simulink model "k1visbs_oktm_20161207"  (Simulink 8.5)
settings: Solver=ode45  StartTime=0.0  StopTime=10.0  RelTol=1e-3
undefined symbols (not defined in the file): AC, FOUROSEM_OPLEV_DAMP_MASTER, SIXOSEM_F_STAGE_MASTER, SIXOSEM_F_WD_AC_MASTER
libraries: cdsEpicsOut x82, cdsFilt x57, cdsTP x36, cdsFiltCtrl x16, VIS_LIB x14, cdsMuxMatrix x13, cdsEpicsIn x10, cdsRms x6, STATE_BIO_MASTER x4, cdsEpicsBinIn x4, lockin x4, cdsFunctionCall x4
(part 1 of 8)
settings Model: Creator=keiko  LastModifiedBy=controls
settings DataIOCC: SignalLoggingSaveFormat=Dataset
settings OptimizationCC: ExpressionDepthLimit=128
settings DebuggingCC: UnderspecifiedInitializationDetection=Simplified  MergeDetectMultiDrivingBlocksExec=error  SolverPrmCheckMsg=warning  FcnCallInpInsideContextMsg=EnableAllAsError  StateNameClashWarn=none
settings GRTTargetCC: CombineOutputUpdateFcns=on  GRTInterface=off

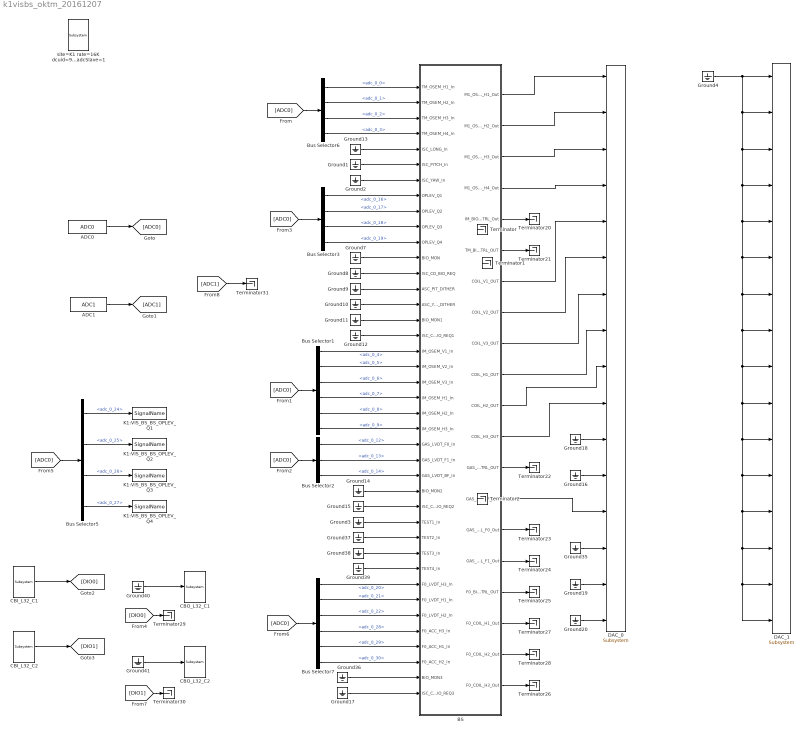
== system k1visbs_oktm_20161207 ==
  ADC0 : cdsAdcx0/ADC0  Tag=cdsAdc  Description=|
      | type-GSC_16AI64SSA
      | card_num=0
      settings: AttributesFormatString=%<Description>\n%<Tag>
  ADC1 : cdsAdcx1/ADC1  Tag=cdsAdc  Description=|
      | type-GSC_16AI64SSA
      | card_num=1
      settings: AttributesFormatString=%<Description>\n%<Tag>
  BS : Subsystem  Description=TYPEB MASTER  AncestorBlock=TYPEB_MASTER/TYPEB MASTER
      settings: AttributesFormatString=%<Description>
  Bus Selector1 : BusSelector  Description=ADC Selector  OutputSignals=adc_0_4,adc_0_5,adc_0_6,adc_0_7,adc_0_8,adc_0_9
      settings: AttributesFormatString=%<Description>
  Bus Selector2 : BusSelector  Description=ADC Selector  OutputSignals=adc_0_12,adc_0_13,adc_0_14
      settings: AttributesFormatString=%<Description>
  Bus Selector3 : BusSelector  Description=ADC Selector  OutputSignals=adc_0_16,adc_0_17,adc_0_18,adc_0_19
      settings: AttributesFormatString=%<Description>
  Bus Selector5 : BusSelector  Description=ADC Selector  OutputSignals=adc_0_24,adc_0_25,adc_0_26,adc_0_27
      settings: AttributesFormatString=%<Description>
  Bus Selector6 : BusSelector  Description=ADC Selector  OutputSignals=adc_0_0,adc_0_1,adc_0_2,adc_0_3
      settings: AttributesFormatString=%<Description>
  Bus Selector7 : BusSelector  Description=ADC Selector  OutputSignals=adc_0_20,adc_0_21,adc_0_22,adc_0_28,adc_0_29,adc_0_30
      settings: AttributesFormatString=%<Description>
  CBI_L32_C1 : cdsCDI64/Subsystem  Tag=cdsCDI64  Description=card_num=0
      settings: AttributesFormatString=%<Tag>\n%<Description>
  CBI_L32_C2 : cdsCDI64/Subsystem  Tag=cdsCDI64  Description=card_num=2
      settings: AttributesFormatString=%<Tag>\n%<Description>
  CBO_L32_C1 : cdsCDO64/Subsystem  Tag=cdsCDO64  Description=card_num=0
      settings: AttributesFormatString=%<Tag>\n%<Description>
  CBO_L32_C2 : cdsCDO64/Subsystem  Tag=cdsCDO64  Description=card_num=2
      settings: AttributesFormatString=%<Tag>\n%<Description>
  DAC_0 : dac/Subsystem  Description=|
      | type=GSC_16AO16,
      | card_num=0
      settings: AttributesFormatString=%<Description>
  DAC_1 : dac/Subsystem  Description=|
      | type=GSC_16AO16,
      | card_num=1
      settings: AttributesFormatString=%<Description>
  Ground{1..4,7..20,35..41} (25 alike) : Ground
  K1:VIS_BS_BS_OPLEV_Q{1..4} (4 alike) : cdsIPCx/SignalName  Tag=cdsIPCx_PCIE  Description=Inter-Process Communication via PCI Express network.
      settings: AttributesFormatString=%<Tag>
  Terminator{,1..2,20..31} (15 alike) : Terminator
  site=K1 rate=16K dcuid=96 host=k1pr2 specific_cpu=4 adcSlave=1 : cdsParameters/Subsystem  Tag=cdsParameters  Description=|
      | Purpose:                                                                                                                                                                                                                                
      | Provide system parameters to the FE code generator to properly configure the generated EPICS names, rep rate of the FE controller, and the Data Acquisition node ID for proper storage of data from this FE controller.                 
      |                                                                                                                                                                                                                                         
      | Useage:                                                                                                                                                                                                                                 
      | The part NAME field is used to identify the FE parameters. It must be of the form:                                                                                                                                                      
      | site=                                                                                                                                                                                                                                   
      | rate=                                                                                                                                                                                                                                   
      | dcuid=                                                                                                                                                                                                                                  
      |                                                                                                                                                                                                                                         
      | Where:                                                                                                                                                                                                                                  
      | site= argument may be H1, H2, L1, M1, G1, either as a single argument or multiple, for example site=H1,H2. These are the only names allowed. These will become the first two characters of all EPICS and signal names (for example G1:).
      |                                                                                                                                                                                                                                         
      | rate= may be 2K, 16K, 32K, or 64K                                                                                                                                                                                                       
      |                                                                                                                                                                                                                                         
      | dcuid= is site specific ie it must be unique at each site.
      settings: AttributesFormatString=%<Tag>
  wires:
  ADC0/1 -> [ADC0]
  [ADC0] -> Bus Selector6/1
  [ADC0] -> Bus Selector1/1
  Bus Selector6/1 -> BS/1(TM_OSEM_H1_In)  "<adc_0_0>"
  Bus Selector6/2 -> BS/2(TM_OSEM_H2_In)  "<adc_0_1>"
  Bus Selector6/3 -> BS/3(TM_OSEM_H3_In)  "<adc_0_2>"
  Bus Selector6/4 -> BS/4(TM_OSEM_H4_In)  "<adc_0_3>"
  Bus Selector3/4 -> BS/11(OPLEV_Q4)  "<adc_0_19>"
  Ground11/1 -> BS/16(BIO_MON1)
  Ground7/1 -> BS/12(BIO_MON)
  Ground2/1 -> BS/7(ISC_YAW_In)
  Ground8/1 -> BS/13(ISC_CD_BIO_REQ)
  Ground1/1 -> BS/6(ISC_PITCH_In)
  Ground12/1 -> BS/17(ISC_CD_BIO_REQ1)
  Ground13/1 -> BS/5(ISC_LONG_In)
  Bus Selector3/1 -> BS/8(OPLEV_Q1)  "<adc_0_16>"
  Bus Selector3/3 -> BS/10(OPLEV_Q3)  "<adc_0_18>"
  Bus Selector3/2 -> BS/9(OPLEV_Q2)  "<adc_0_17>"
  Ground10/1 -> BS/15(ASC_YAW_DITHER)
  Ground9/1 -> BS/14(ASC_PIT_DITHER)
  Bus Selector1/1 -> BS/18(IM_OSEM_V1_In)  "<adc_0_4>"
  Bus Selector1/2 -> BS/19(IM_OSEM_V2_In)  "<adc_0_5>"
  Bus Selector1/3 -> BS/20(IM_OSEM_V3_In)  "<adc_0_6>"
  Bus Selector1/4 -> BS/21(IM_OSEM_H1_In)  "<adc_0_7>"
  Bus Selector1/5 -> BS/22(IM_OSEM_H2_In)  "<adc_0_8>"
  Bus Selector1/6 -> BS/23(IM_OSEM_H3_In)  "<adc_0_9>"
  Ground14/1 -> BS/27(BIO_MON2)
  Ground15/1 -> BS/28(ISC_CD_BIO_REQ2)
  [ADC0] -> Bus Selector2/1
  Bus Selector2/1 -> BS/24(GAS_LVDT_F0_In)  "<adc_0_12>"
  [ADC0] -> Bus Selector3/1
  Ground3/1 -> BS/29(TEST1_In)
  [ADC0] -> Bus Selector5/1
  Bus Selector5/1 -> K1:VIS_BS_BS_OPLEV_Q1/1  "<adc_0_24>"
  Bus Selector5/2 -> K1:VIS_BS_BS_OPLEV_Q2/1  "<adc_0_25>"
  Bus Selector5/3 -> K1:VIS_BS_BS_OPLEV_Q3/1  "<adc_0_26>"
  Bus Selector5/4 -> K1:VIS_BS_BS_OPLEV_Q4/1  "<adc_0_27>"
  BS/1(M1_OSEM_H1_Out) -> DAC_0/1
  BS/2(M1_OSEM_H2_Out) -> DAC_0/2
  BS/3(M1_OSEM_H3_Out) -> DAC_0/3
  BS/4(M1_OSEM_H4_Out) -> DAC_0/4
  BS/5(IM_BIO_CTRL_Out) -> Terminator20/1
  BS/6(TM_BIO_CTRL_OUT) -> Terminator21/1
  Ground18/1 -> DAC_0/11
  Ground16/1 -> DAC_0/12
  Ground35/1 -> DAC_0/14
  Ground19/1 -> DAC_0/15
  Ground20/1 -> DAC_0/16
  BS/13(GAS_BIO_CTRL_OUT) -> Terminator22/1
  BS/14(GAS_COIL_BF_Out) -> DAC_0/13
  BS/10(COIL_H1_OUT) -> DAC_0/8
  BS/7(COIL_V1_OUT) -> DAC_0/5
  BS/9(COIL_V3_OUT) -> DAC_0/7
  BS/8(COIL_V2_OUT) -> DAC_0/6
  BS/11(COIL_H2_OUT) -> DAC_0/9
  BS/12(COIL_H3_OUT) -> DAC_0/10
  Ground17/1 -> BS/40(ISC_CD_BIO_REQ3)
  Bus Selector2/2 -> BS/25(GAS_LVDT_F1_In)  "<adc_0_13>"
  Bus Selector2/3 -> BS/26(GAS_LVDT_BF_In)  "<adc_0_14>"
  BS/15(GAS_COIL_F0_Out) -> Terminator23/1
  BS/16(GAS_COIL_F1_Out) -> Terminator24/1
  BS/17(F0_BIO_CTRL_OUT) -> Terminator25/1
  BS/20(F0_COIL_H3_Out) -> Terminator26/1
  BS/18(F0_COIL_H1_Out) -> Terminator27/1
  BS/19(F0_COIL_H2_Out) -> Terminator28/1
  [ADC0] -> Bus Selector7/1
  Ground36/1 -> BS/39(BIO_MON3)
  Ground37/1 -> BS/30(TEST2_In)
  Ground38/1 -> BS/31(TEST3_In)
  Ground39/1 -> BS/32(TEST4_In)
  Bus Selector7/1 -> BS/33(F0_LVDT_H3_In)  "<adc_0_20>"
  Bus Selector7/5 -> BS/37(F0_ACC_H1_In)  "<adc_0_29>"
  Bus Selector7/6 -> BS/38(F0_ACC_H2_In)  "<adc_0_30>"
  Bus Selector7/3 -> BS/35(F0_LVDT_H2_In)  "<adc_0_22>"
  Bus Selector7/2 -> BS/34(F0_LVDT_H1_In)  "<adc_0_21>"
  Bus Selector7/4 -> BS/36(F0_ACC_H3_In)  "<adc_0_28>"
  ADC1/1 -> [ADC1]
  CBI_L32_C1/1 -> [DIO0]
  CBI_L32_C2/1 -> [DIO1]
  Ground40/1 -> CBO_L32_C1/1
  Ground41/1 -> CBO_L32_C2/1
  [DIO0] -> Terminator29/1
  [DIO1] -> Terminator30/1
  [ADC1] -> Terminator31/1
  Ground4/1 -> DAC_1/6, DAC_1/16, DAC_1/15, DAC_1/14, DAC_1/13, DAC_1/12, DAC_1/11, DAC_1/10, DAC_1/9, DAC_1/8, DAC_1/7, DAC_1/5, DAC_1/4, DAC_1/3, DAC_1/2, DAC_1/1

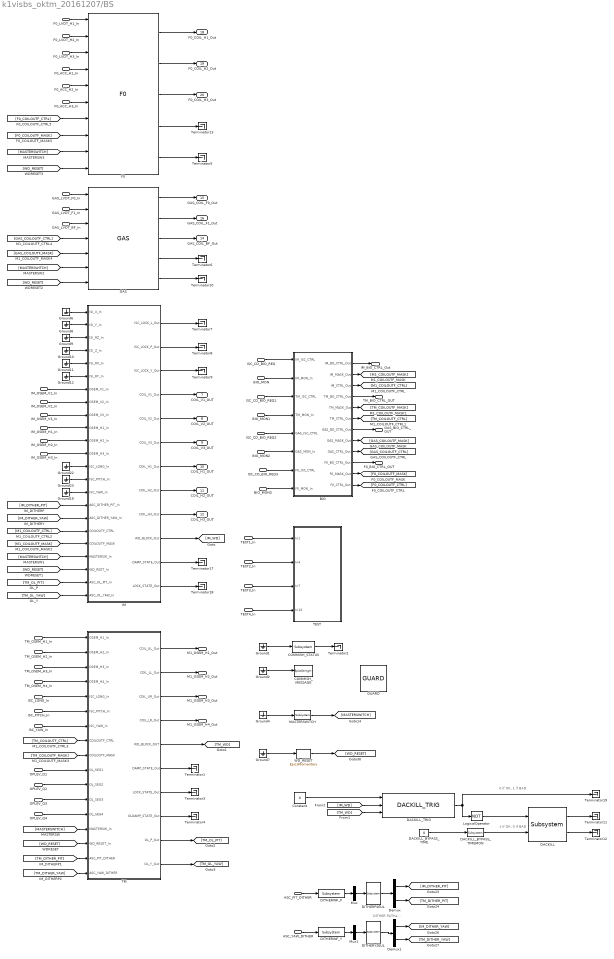
== system k1visbs_oktm_20161207/BS ==
  note: 1 if OK, 0 if BAD
  note: 0 if OK, 1 if BAD
  note: DITHER PATHs
      |
      |
      |
      |
      |
      |
      |
      |
      |
      |
      |
      |
      |
      |
      | .                                                                                                      .
  TM_OSEM_H1_In : Inport
  TM_OSEM_H2_In : Inport  Port=2
  TM_OSEM_H3_In : Inport  Port=3
  TM_OSEM_H4_In : Inport  Port=4
  ISC_LONG_In : Inport  Port=5
  ISC_PITCH_In : Inport  Port=6
  ISC_YAW_In : Inport  Port=7
  OPLEV_Q1 : Inport  Port=8
  OPLEV_Q2 : Inport  Port=9
  OPLEV_Q3 : Inport  Port=10
  OPLEV_Q4 : Inport  Port=11
  BIO_MON : Inport  Port=12
  ISC_CD_BIO_REQ : Inport  Port=13
  ASC_PIT_DITHER : Inport  Port=14
  ASC_YAW_DITHER : Inport  Port=15
  BIO_MON1 : Inport  Port=16
  ISC_CD_BIO_REQ1 : Inport  Port=17
  IM_OSEM_V1_In : Inport  Port=18
  IM_OSEM_V2_In : Inport  Port=19
  IM_OSEM_V3_In : Inport  Port=20
  IM_OSEM_H1_In : Inport  Port=21
  IM_OSEM_H2_In : Inport  Port=22
  IM_OSEM_H3_In : Inport  Port=23
  GAS_LVDT_F0_In : Inport  Port=24
  GAS_LVDT_F1_In : Inport  Port=25
  GAS_LVDT_BF_In : Inport  Port=26
  BIO_MON2 : Inport  Port=27
  ISC_CD_BIO_REQ2 : Inport  Port=28
  TEST1_In : Inport  Port=29
  TEST2_In : Inport  Port=30
  TEST3_In : Inport  Port=31
  TEST4_In : Inport  Port=32
  F0_LVDT_H3_In : Inport  Port=33
  F0_LVDT_H1_In : Inport  Port=34
  F0_LVDT_H2_In : Inport  Port=35
  F0_ACC_H3_In : Inport  Port=36
  F0_ACC_H1_In : Inport  Port=37
  F0_ACC_H2_In : Inport  Port=38
  BIO_MON3 : Inport  Port=39
  ISC_CD_BIO_REQ3 : Inport  Port=40
  BIO : Subsystem
  COMMISH_MESSAGE : cdsEpicsStringIn/EpicsStringIn  Tag=cdsEpicsStringIn  Description=cdsEpicsStringIn
      settings: AttributesFormatString=%<Tag>
  COMMISH_STATUS : cdsEpicsBinIn/Subsystem  Tag=cdsEpicsBinIn  Description=|
      | Purpose:                                                                            
      | Create an EPICS binary (0 or 1) input channel to the FE realtime controls.          
      |                                                                                     
      | Operation:                                                                          
      | Outputs value from an EPICS ai record. Value is binary input (bi Epics record type).
      |                                                                                     
      | Usage:                                                                              
      | Name the part with the desired EPICS channel name.
      settings: AttributesFormatString=%<Tag>
  Constant : Constant  Value=0
  DACKILL : cdsDacKill/Subsystem  Description=cdsDacKill
      settings: AttributesFormatString=%<Description>
  DACKILL_BYPASS_TIME : Constant  Value=0
  DACKILL_BYPASS_TIMEMON : cdsEpicsOut/Subsystem  Tag=cdsEpicsOutput  Description=|
      | Purpose:                                          
      | Output a FE signal to an EPICS channel.           
      |                                                   
      | Operation:                                        
      | Takes input value and passes it to EPICS record.  
      |                                                   
      | Usage:                                            
      | Name the part with the desired EPICS rrecord name.
      settings: AttributesFormatString=%<Tag>
  DACKILL_TRIG : VIS_LIB/DACKILL_TRIG
  DITHERINF_P : cdsFilt/Subsystem  Tag=cdsFilt  Description=|
      | Purpose:                                                                                                                                                                                                                                  
      | Standard CDS IIR filter module.                                                                                                                                                                                                           
      |                                                                                                                                                                                                                                           
      | Operation:                                                                                                                                                                                                                                
      | Consists of 10 second order section IIR filters, plus a ramped gain stage. In FE code, also provides pre-defined test points and excitation channel inputs. The filter coefficients are defined in the LIGO system using the 'foton' tool.
      |                                                                                                                                                                                                                                           
      | Usage:                                                                                                                                                                                                                                    
      | Name the part with the desired filter module name.
      settings: AttributesFormatString=%<Tag>
  DITHERINF_Y : cdsFilt/Subsystem  Tag=cdsFilt  Description=|
      | Purpose:                                                                                                                                                                                                                                  
      | Standard CDS IIR filter module.                                                                                                                                                                                                           
      |                                                                                                                                                                                                                                           
      | Operation:                                                                                                                                                                                                                                
      | Consists of 10 second order section IIR filters, plus a ramped gain stage. In FE code, also provides pre-defined test points and excitation channel inputs. The filter coefficients are defined in the LIGO system using the 'foton' tool.
      |                                                                                                                                                                                                                                           
      | Usage:                                                                                                                                                                                                                                    
      | Name the part with the desired filter module name.
      settings: AttributesFormatString=%<Tag>
  DITHERP2EUL : cdsMuxMatrix/Subsystem  Tag=cdsMuxMatrix  Description=Any size matrix. Inputs and outputs must be connected using Mux and Demux parts.
      settings: AttributesFormatString=%<Tag>
  DITHERY2EUL : cdsMuxMatrix/Subsystem  Tag=cdsMuxMatrix  Description=Any size matrix. Inputs and outputs must be connected using Mux and Demux parts.
      settings: AttributesFormatString=%<Tag>
  Demux : Demux  Outputs=2
  Demux1 : Demux  Outputs=2
  F0 : F0_MASTER/F0
  GAS : GAS_TYPEB_MASTER/GAS  Tag=GAS_TYPEB_MASTER  Description=GAS_TYPEB_MASTER
  GUARD : ISC_common/GUARD
  Ground{1..2,4,6..12,19,22..23} (13 alike) : Ground
  IM : Subsystem  Description=SIXOSEMSTAGE_FACE_MASTER  AncestorBlock=SIXOSEM_F_STAGE_MASTER/SIXOSEM_F_STAGE_MASTER
  LogicalOperator : Logic  Operator=NOT  AllPortsSameDT=off  OutDataTypeStr=boolean
  MASTERSWITCH : cdsEpicsBinIn/Subsystem  Tag=cdsEpicsBinIn  Description=|
      | Purpose:                                                                            
      | Create an EPICS binary (0 or 1) input channel to the FE realtime controls.          
      |                                                                                     
      | Operation:                                                                          
      | Outputs value from an EPICS ai record. Value is binary input (bi Epics record type).
      |                                                                                     
      | Usage:                                                                              
      | Name the part with the desired EPICS channel name.
      settings: AttributesFormatString=%<Tag>
  Mux : Mux  Inputs=1
  Mux1 : Mux  Inputs=1
  TEST : Subsystem
  TM : Subsystem  AncestorBlock=FOUROSEM_OPLEV_DAMP_MASTER/FOUROSEM_OPLEV_DAMP_MASTER
  Terminator{1..13,17..19} (16 alike) : Terminator
  WD_RESET : cdsEpicsMomentary/EpicsMomentary  Tag=cdsEpicsMomentary
      settings: AttributesFormatString=%<Tag>
  M1_OSEM_H1_Out : Outport
  M1_OSEM_H2_Out : Outport  Port=2
  M1_OSEM_H3_Out : Outport  Port=3
  M1_OSEM_H4_Out : Outport  Port=4
  IM_BIO_CTRL_Out : Outport  Port=5
  TM_BIO_CTRL_OUT : Outport  Port=6
  COIL_V1_OUT : Outport  Port=7
  COIL_V2_OUT : Outport  Port=8
  COIL_V3_OUT : Outport  Port=9
  COIL_H1_OUT : Outport  Port=10
  COIL_H2_OUT : Outport  Port=11
  COIL_H3_OUT : Outport  Port=12
  GAS_BIO_CTRL_OUT : Outport  Port=13
  GAS_COIL_BF_Out : Outport  Port=14
  GAS_COIL_F0_Out : Outport  Port=15
  GAS_COIL_F1_Out : Outport  Port=16
  F0_BIO_CTRL_OUT : Outport  Port=17
  F0_COIL_H1_Out : Outport  Port=18
  F0_COIL_H2_Out : Outport  Port=19
  F0_COIL_H3_Out : Outport  Port=20
  wires:
  F0_ACC_H2_In/1 -> F0/5
  F0_LVDT_H3_In/1 -> F0/3
  F0_LVDT_H1_In/1 -> F0/1
  F0_ACC_H1_In/1 -> F0/4
  F0_LVDT_H2_In/1 -> F0/2
  F0_ACC_H3_In/1 -> F0/6
  GAS/2 -> GAS_COIL_F1_Out/1
  GAS/1 -> GAS_COIL_F0_Out/1
  GAS_LVDT_F0_In/1 -> GAS/1
  GAS_LVDT_F1_In/1 -> GAS/2
  TM/10(OL_Y_Out) -> [TM_OL_YAW]
  TM/9(OL_P_Out) -> [TM_OL_PIT]
  [TM_OL_YAW] -> IM/23(ASC_OL_YAW_In)
  [TM_OL_PIT] -> IM/22(ASC_OL_PIT_In)
  [WD_RESET] -> IM/21(WD_RSET_In)
  [MASTERSWITCH] -> IM/20(MASTERSW_In)
  [M1_COILOUTF_MASK] -> IM/19(COILOUTF_MASK)
  [IM_DITHER_YAW] -> IM/17(ASC_DITHER_YAW_In)
  [IM_DITHER_PIT] -> IM/16(ASC_DITHER_PIT_In)
  [M1_COILOUTF_CTRL] -> IM/18(COILOUTF_CTRL)
  [IM_WD] -> DACKILL_TRIG/2
  DACKILL/2 -> Terminator12/1
  DACKILL/1 -> Terminator11/1
  DACKILL_BYPASS_TIME/1 -> DACKILL_BYPASS_TIMEMON/1
  DACKILL_BYPASS_TIMEMON/1 -> DACKILL/2
  LogicalOperator/1 -> DACKILL/1
  DACKILL_TRIG/1 -> LogicalOperator/1, Terminator19/1
  Constant/1 -> DACKILL_TRIG/1
  [TM_WD] -> DACKILL_TRIG/3
  TM/1(COIL_UL_Out) -> M1_OSEM_H1_Out/1
  TEST4_In/1 -> TEST/4(In10)
  TEST1_In/1 -> TEST/1(In1)
  TEST2_In/1 -> TEST/2(In4)
  TEST3_In/1 -> TEST/3(In7)
  GAS/5 -> Terminator10/1
  GAS/4 -> Terminator6/1
  GAS/3 -> GAS_COIL_BF_Out/1
  [WD_RESET] -> GAS/7
  [MASTERSWITCH] -> GAS/6
  [GAS_COILOUTF_MASK] -> GAS/5
  BIO_MON2/1 -> BIO/6(GAS_MON_In)
  ISC_CD_BIO_REQ2/1 -> BIO/5(GAS_ISC_CTRL)
  BIO/9(GAS_CTRL_Out) -> [GAS_COILOUTF_CTRL]
  BIO/8(GAS_MASK_Out) -> [GAS_COILOUTF_MASK]
  BIO/7(GAS_BO_CTRL_Out) -> GAS_BIO_CTRL_OUT/1
  [GAS_COILOUTF_CTRL] -> GAS/4
  GAS_LVDT_BF_In/1 -> GAS/3
  IM/9(COIL_H3_Out) -> COIL_H3_OUT/1
  IM/8(COIL_H2_Out) -> COIL_H2_OUT/1
  IM/7(COIL_H1_Out) -> COIL_H1_OUT/1
  IM/6(COIL_V3_Out) -> COIL_V3_OUT/1
  IM/5(COIL_V2_Out) -> COIL_V2_OUT/1
  IM/4(COIL_V1_Out) -> COIL_V1_OUT/1
  IM_OSEM_H1_In/1 -> IM/10(OSEM_H1_In)
  IM_OSEM_H2_In/1 -> IM/11(OSEM_H2_In)
  IM_OSEM_H3_In/1 -> IM/12(OSEM_H3_In)
  IM_OSEM_V1_In/1 -> IM/7(OSEM_V1_In)
  IM_OSEM_V2_In/1 -> IM/8(OSEM_V2_In)
  IM_OSEM_V3_In/1 -> IM/9(OSEM_V3_In)
  IM/12(LOCK_STATE_Out) -> Terminator18/1
  IM/3(ISC_LOCK_Y_Out) -> Terminator9/1
  IM/2(ISC_LOCK_P_Out) -> Terminator8/1
  IM/11(DAMP_STATE_Out) -> Terminator17/1
  IM/10(WD_BLOCK_Out) -> [IM_WD]
  IM/1(ISC_LOCK_L_Out) -> Terminator7/1
  Ground19/1 -> IM/15(ISC_YAW_In)
  Ground23/1 -> IM/14(ISC_PITCH_In)
  Ground12/1 -> IM/6(ISI_RY_In)
  Ground10/1 -> IM/4(ISI_Z_In)
  Ground22/1 -> IM/13(ISC_LONG_In)
  Ground8/1 -> IM/2(ISI_Y_In)
  Ground6/1 -> IM/1(ISI_X_In)
  Ground11/1 -> IM/5(ISI_RX_In)
  Ground9/1 -> IM/3(ISI_RZ_In)
  [TM_DITHER_YAW] -> TM/17(ASC_YAW_DITHER)
  [TM_DITHER_PIT] -> TM/16(ASC_PIT_DITHER)
  DITHERINF_Y/1 -> Mux1/1
  DITHERINF_P/1 -> Mux/1
  Demux1/2 -> [TM_DITHER_YAW]
  Demux1/1 -> [IM_DITHER_YAW]
  Demux/2 -> [TM_DITHER_PIT]
  Demux/1 -> [IM_DITHER_PIT]
  DITHERY2EUL/1 -> Demux1/1
  Mux1/1 -> DITHERY2EUL/1
  ASC_PIT_DITHER/1 -> DITHERINF_P/1
  DITHERP2EUL/1 -> Demux/1
  Mux/1 -> DITHERP2EUL/1
  ASC_YAW_DITHER/1 -> DITHERINF_Y/1
  Ground1/1 -> COMMISH_STATUS/1
  COMMISH_STATUS/1 -> Terminator2/1
  Ground2/1 -> COMMISH_MESSAGE/1
  TM_OSEM_H1_In/1 -> TM/1(OSEM_H1_In)
  TM_OSEM_H2_In/1 -> TM/2(OSEM_H2_In)
  TM_OSEM_H3_In/1 -> TM/3(OSEM_H3_In)
  TM_OSEM_H4_In/1 -> TM/4(OSEM_H4_In)
  ISC_LONG_In/1 -> TM/5(ISC_LONG_In)
  TM/5(WD_BLOCK_OUT) -> [TM_WD]
  BIO/3(IM_CTRL_Out) -> [M1_COILOUTF_CTRL]
  BIO/2(IM_MASK_Out) -> [M1_COILOUTF_MASK]
  BIO/1(IM_BO_CTRL_Out) -> IM_BIO_CTRL_Out/1
  TM/2(COIL_LL_Out) -> M1_OSEM_H2_Out/1
  TM/3(COIL_UR_Out) -> M1_OSEM_H3_Out/1
  TM/4(COIL_LR_Out) -> M1_OSEM_H4_Out/1
  BIO_MON/1 -> BIO/2(IM_MON_In)
  ISC_CD_BIO_REQ/1 -> BIO/1(IM_ISC_CTRL)
  MASTERSWITCH/1 -> [MASTERSWITCH]
  Ground4/1 -> MASTERSWITCH/1
  OPLEV_Q1/1 -> TM/10(OL_SEG1)
  OPLEV_Q2/1 -> TM/11(OL_SEG2)
  OPLEV_Q3/1 -> TM/12(OL_SEG3)
  ISC_PITCH_In/1 -> TM/6(ISC_PITCH_In)
  ISC_YAW_In/1 -> TM/7(ISC_YAW_In)
  OPLEV_Q4/1 -> TM/13(OL_SEG4)
  [MASTERSWITCH] -> TM/14(MASTERSW_In)
  TM/8(OLDAMP_STATE_Out) -> Terminator4/1
  TM/7(LOCK_STATE_Out) -> Terminator3/1
  TM/6(DAMP_STATE_Out) -> Terminator1/1
  Ground7/1 -> WD_RESET/1
  WD_RESET/1 -> [WD_RESET]
  [WD_RESET] -> TM/15(WD_RESET_In)
  BIO_MON1/1 -> BIO/4(TM_MON_In)
  ISC_CD_BIO_REQ1/1 -> BIO/3(TM_ISC_CTRL)
  BIO/5(TM_MASK_Out) -> [TM_COILOUTF_MASK]
  BIO/6(TM_CTRL_Out) -> [TM_COILOUTF_CTRL]
  BIO/4(TM_BO_CTRL_Out) -> TM_BIO_CTRL_OUT/1
  [TM_COILOUTF_CTRL] -> TM/8(COILOUTF_CTRL)
  [TM_COILOUTF_MASK] -> TM/9(COILOUTF_MASK)
  [MASTERSWITCH] -> F0/9
  [WD_RESET] -> F0/10
  BIO/11(F0_MASK_Out) -> [F0_COILOUTF_MASK]
  BIO/12(F0_CTRL_Out) -> [F0_COILOUTF_CTRL]
  BIO/10(F0_BO_CTRL_Out) -> F0_BIO_CTRL_OUT/1
  BIO_MON3/1 -> BIO/8(F0_MON_In)
  ISC_CD_BIO_REQ3/1 -> BIO/7(F0_ISC_CTRL)
  [F0_COILOUTF_CTRL] -> F0/7
  [F0_COILOUTF_MASK] -> F0/8
  F0/5 -> Terminator5/1
  F0/4 -> Terminator13/1
  F0/3 -> F0_COIL_H3_Out/1
  F0/2 -> F0_COIL_H2_Out/1
  F0/1 -> F0_COIL_H1_Out/1

== system k1visbs_oktm_20161207/BS/BIO ==
  note: 12 Bit Word
  note: 12 Bit Word
  note: 12 Bit Word
  note: 12 Bit Word
  note: 12 Bit Word
  note: 12 Bit Word
  note: 12 Bit Word
  note: 12 Bit Word
  IM_ISC_CTRL : Inport
  IM_MON_In : Inport  Port=2
  TM_ISC_CTRL : Inport  Port=3
  TM_MON_In : Inport  Port=4
  GAS_ISC_CTRL : Inport  Port=5
  GAS_MON_In : Inport  Port=6
  F0_ISC_CTRL : Inport  Port=7
  F0_MON_In : Inport  Port=8
  F0 : STATE_BIO_MASTER/TACQ_BIO_MASTER
  GAS : STATE_BIO_MASTER/TACQ_BIO_MASTER
  IM : STATE_BIO_MASTER/TOP_BIO_MASTER
  TM : STATE_BIO_MASTER/TACQ_BIO_MASTER
  IM_BO_CTRL_Out : Outport
  IM_MASK_Out : Outport  Port=2
  IM_CTRL_Out : Outport  Port=3
  TM_BO_CTRL_Out : Outport  Port=4
  TM_MASK_Out : Outport  Port=5
  TM_CTRL_Out : Outport  Port=6
  GAS_BO_CTRL_Out : Outport  Port=7
  GAS_MASK_Out : Outport  Port=8
  GAS_CTRL_Out : Outport  Port=9
  F0_BO_CTRL_Out : Outport  Port=10
  F0_MASK_Out : Outport  Port=11
  F0_CTRL_Out : Outport  Port=12
  wires:
  GAS/2 -> GAS_CTRL_Out/1
  GAS/1 -> GAS_MASK_Out/1
  GAS/3 -> GAS_BO_CTRL_Out/1
  GAS_MON_In/1 -> GAS/2
  GAS_ISC_CTRL/1 -> GAS/1
  IM/2 -> IM_CTRL_Out/1
  IM/1 -> IM_MASK_Out/1
  IM/3 -> IM_BO_CTRL_Out/1
  IM_MON_In/1 -> IM/2
  IM_ISC_CTRL/1 -> IM/1
  TM/2 -> TM_CTRL_Out/1
  TM/1 -> TM_MASK_Out/1
  TM/3 -> TM_BO_CTRL_Out/1
  TM_MON_In/1 -> TM/2
  TM_ISC_CTRL/1 -> TM/1
  F0/2 -> F0_CTRL_Out/1
  F0/1 -> F0_MASK_Out/1
  F0/3 -> F0_BO_CTRL_Out/1
  F0_MON_In/1 -> F0/2
  F0_ISC_CTRL/1 -> F0/1

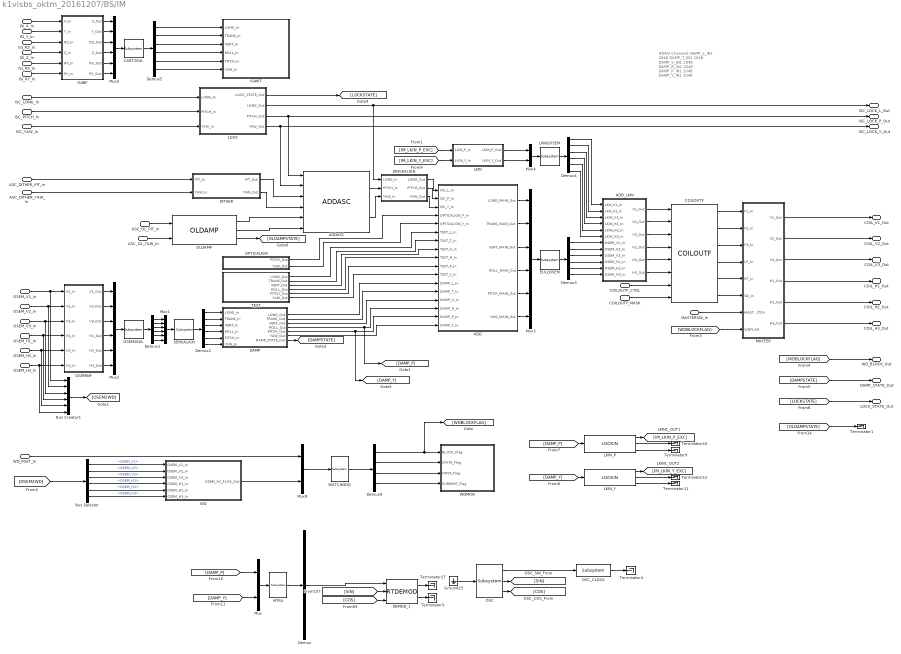
== system k1visbs_oktm_20161207/BS/IM ==
  note: #DAQ Channels
      | DAMP_L_IN1 2048
      | DAMP_T_IN1 2048
      | DAMP_V_IN1 2048
      | DAMP_R_IN1 2048
      | DAMP_P_IN1 2048
      | DAMP_Y_IN1 2048
  ISI_X_In : Inport
  ISI_Y_In : Inport  Port=2
  ISI_RZ_In : Inport  Port=3
  ISI_Z_In : Inport  Port=4
  ISI_RX_In : Inport  Port=5
  ISI_RY_In : Inport  Port=6
  OSEM_V1_In : Inport  Port=7
  OSEM_V2_In : Inport  Port=8
  OSEM_V3_In : Inport  Port=9
  OSEM_H1_In : Inport  Port=10
  OSEM_H2_In : Inport  Port=11
  OSEM_H3_In : Inport  Port=12
  ISC_LONG_In : Inport  Port=13
  ISC_PITCH_In : Inport  Port=14
  ISC_YAW_In : Inport  Port=15
  ASC_DITHER_PIT_In : Inport  Port=16
  ASC_DITHER_YAW_In : Inport  Port=17
  COILOUTF_CTRL : Inport  Port=18
  COILOUTF_MASK : Inport  Port=19
  MASTERSW_In : Inport  Port=20
  WD_RSET_In : Inport  Port=21
  ASC_OL_PIT_In : Inport  Port=22
  ASC_OL_YAW_In : Inport  Port=23
  ADD : Subsystem
  ADDASC : VIS_LIB/ADDASC
  ADD_LKIN : Subsystem
  Bus Creator1 : BusCreator  Inputs='OSEM_V1','OSEM_V2','OSEM_V3','OSEM_H1','OSEM_H2','OSEM_H3'
  Bus Selector : BusSelector  OutputSignals=OSEM_V1,OSEM_V2,OSEM_V3,OSEM_H1,OSEM_H2,OSEM_H3
  CART2EUL : cdsMuxMatrix/Subsystem  Tag=cdsMuxMatrix  Description=Any size matrix. Inputs and outputs must be connected using Mux and Demux parts.
      settings: AttributesFormatString=%<Tag>
  COILOUTF : SIXOSEM_F_COILOUTF_MASTER/COILOUTF
  DAMP : Subsystem
  DEMOD_1 : rtdemod/RTDEMOD  Tag=top_names
  DITHER : Subsystem
  DRIVEALIGN : Subsystem
  Demux : Demux  Outputs=1
  Demux{1..5} (5 alike) : Demux  Outputs=6
  Demux9 : Demux
  EUL2OSEM : cdsMuxMatrix/Subsystem  Tag=cdsMuxMatrix  Description=Any size matrix. Inputs and outputs must be connected using Mux and Demux parts.
      settings: AttributesFormatString=%<Tag>
  Ground23 : Ground
  ISIINF : Subsystem
  ISIWIT : Subsystem
  LKIN : Subsystem
  LKIN2OSEM : cdsMuxMatrix/Subsystem  Tag=cdsMuxMatrix  Description=Any size matrix. Inputs and outputs must be connected using Mux and Demux parts.
      settings: AttributesFormatString=%<Tag>
  LKIN_P : lockin/LOCKIN  Description=ADL=LOCKIN.adl
      settings: AttributesFormatString=%<Tag>
  LKIN_Y : lockin/LOCKIN  Description=ADL=LOCKIN.adl
      settings: AttributesFormatString=%<Tag>
  LOCK : Subsystem
  MASTER : Subsystem
  MTRX : cdsMuxMatrix/Subsystem  Tag=cdsMuxMatrix  Description=Any size matrix. Inputs and outputs must be connected using Mux and Demux parts.
      settings: AttributesFormatString=%<Tag>
  Mux : Mux  Inputs=2
  Mux{1..3,5} (4 alike) : Mux  Inputs=6
  Mux4 : Mux  Inputs=2
  Mux9 : Mux  Inputs=2
  OLDAMP : VIS_LIB/OLDAMP
  OPTICALIGN : Subsystem
  OSC : cdsOsc/Subsystem  Tag=cdsOsc  Description=Oscillator
      settings: AttributesFormatString=%<Tag>
  OSC_CLOCK : cdsEpicsOut/Subsystem  Tag=cdsEpicsOutput  Description=|
      | Purpose:                                          
      | Output a FE signal to an EPICS channel.           
      |                                                   
      | Operation:                                        
      | Takes input value and passes it to EPICS record.  
      |                                                   
      | Usage:                                            
      | Name the part with the desired EPICS rrecord name.
      settings: AttributesFormatString=%<Tag>
  OSEM2EUL : cdsMuxMatrix/Subsystem  Tag=cdsMuxMatrix  Description=Any size matrix. Inputs and outputs must be connected using Mux and Demux parts.
      settings: AttributesFormatString=%<Tag>
  OSEMINF : Subsystem
  SENSALIGN : cdsMuxMatrix/Subsystem  Tag=cdsMuxMatrix  Description=Any size matrix. Inputs and outputs must be connected using Mux and Demux parts.
      settings: AttributesFormatString=%<Tag>
  TEST : Subsystem
  Terminator{1,3..4,9..12,27} (8 alike) : Terminator
  WATCHDOG : cdsFunctionCall/Subsystem  Tag=cdsFunctionCall  Description=inline OSEMWATCHDOG /opt/rtcds/userapps/release/vis/common/src/WATCHDOG.c
      settings: AttributesFormatString=%<Tag>\n%<Description>
  WD : Subsystem
  WDMON : Subsystem
  ISC_LOCK_L_Out : Outport
  ISC_LOCK_P_Out : Outport  Port=2
  ISC_LOCK_Y_Out : Outport  Port=3
  COIL_V1_Out : Outport  Port=4
  COIL_V2_Out : Outport  Port=5
  COIL_V3_Out : Outport  Port=6
  COIL_H1_Out : Outport  Port=7
  COIL_H2_Out : Outport  Port=8
  COIL_H3_Out : Outport  Port=9
  WD_BLOCK_Out : Outport  Port=10
  DAMP_STATE_Out : Outport  Port=11
  LOCK_STATE_Out : Outport  Port=12
  wires:
  [OLDAMPSTATE] -> Terminator1/1
  ASC_OL_PIT_In/1 -> OLDAMP/1
  ASC_OL_YAW_In/1 -> OLDAMP/2
  OLDAMP/1 -> ADDASC/5
  OLDAMP/2 -> ADDASC/6
  OLDAMP/3 -> [OLDAMPSTATE]
  Mux/1 -> MTRX/1
  MTRX/1 -> Demux/1
  Demux/1 -> DEMOD_1/1
  [SIN] -> DEMOD_1/2
  [COS] -> DEMOD_1/3
  DEMOD_1/1 -> Terminator27/1
  DEMOD_1/2 -> Terminator3/1
  Ground23/1 -> OSC/1
  OSC/1 -> OSC_CLOCK/1
  OSC_CLOCK/1 -> Terminator4/1
  OSC/2 -> [SIN]
  OSC/3 -> [COS]
  [DAMP_P] -> Mux/1
  [DAMP_Y] -> Mux/2
  [DAMP_Y] -> LKIN_Y/1
  [DAMP_P] -> LKIN_P/1
  [IM_LKIN_Y_EXC] -> LKIN/2(LKIN_Y_In)
  [IM_LKIN_P_EXC] -> LKIN/1(LKIN_P_In)
  LKIN_Y/3 -> Terminator11/1
  LKIN_Y/2 -> Terminator12/1
  LKIN_Y/1 -> [IM_LKIN_Y_EXC]
  LKIN_P/1 -> [IM_LKIN_P_EXC]
  LKIN_P/3 -> Terminator9/1
  LKIN_P/2 -> Terminator10/1
  DAMP/1(LONG_Out) -> ADD/12(DAMP_L_In)
  DAMP/2(TRANS_Out) -> ADD/13(DAMP_T_In)
  DAMP/3(VERT_Out) -> ADD/14(DAMP_V_In)
  DAMP/4(ROLL_Out) -> ADD/15(DAMP_R_In), [DAMP_P]
  DAMP/5(PITCH_Out) -> ADD/16(DAMP_P_In), [DAMP_Y]
  DAMP/6(YAW_Out) -> ADD/17(DAMP_Y_In)
  TEST/1(LONG_Out) -> ADD/6(TEST_L_In)
  TEST/2(TRANS_Out) -> ADD/7(TEST_T_In)
  TEST/3(VERT_Out) -> ADD/8(TEST_V_In)
  TEST/4(ROLL_Out) -> ADD/9(TEST_R_In)
  TEST/5(PITCH_Out) -> ADD/10(TEST_P_In)
  TEST/6(YAW_Out) -> ADD/11(TEST_Y_In)
  OPTICALIGN/1(PITCH_Out) -> ADD/4(OPTICALIGN_P_In)
  OPTICALIGN/2(YAW_Out) -> ADD/5(OPTICALIGN_Y_In)
  DITHER/1(PIT_Out) -> ADDASC/3
  DITHER/2(YAW_Out) -> ADDASC/4
  ASC_DITHER_PIT_In/1 -> DITHER/1(PIT_In)
  ASC_DITHER_YAW_In/1 -> DITHER/2(YAW_In)
  ADDASC/2 -> DRIVEALIGN/3(YAW_In)
  ADDASC/1 -> DRIVEALIGN/2(PITCH_In)
  DRIVEALIGN/1(LONG_Out) -> ADD/1(ISC_L_In)
  DRIVEALIGN/2(PITCH_Out) -> ADD/2(ISC_P_In)
  DRIVEALIGN/3(YAW_Out) -> ADD/3(ISC_Y_In)
  LOCK/4(YAW_Out) -> ISC_LOCK_Y_Out/1, ADDASC/2
  LOCK/3(PITCH_Out) -> ISC_LOCK_P_Out/1, ADDASC/1
  LOCK/2(LONG_Out) -> ISC_LOCK_L_Out/1, DRIVEALIGN/1(LONG_In)
  WD_RSET_In/1 -> Mux9/1
  WD/1(OSEM_AC_FLAG_Out) -> Mux9/2
  LKIN/2(LKIN_Y_Out) -> Mux4/2
  COILOUTF_CTRL/1 -> COILOUTF/7
  COILOUTF_MASK/1 -> COILOUTF/8
  MASTERSW_In/1 -> MASTER/7(MASTERSWITCH)
  Demux3/6 -> ADD_LKIN/12(OSEM_H3_In)
  Demux3/5 -> ADD_LKIN/11(OSEM_H2_In)
  Demux3/4 -> ADD_LKIN/10(OSEM_H1_In)
  Demux3/3 -> ADD_LKIN/9(OSEM_V3_In)
  Demux3/2 -> ADD_LKIN/8(OSEM_V2_In)
  Demux3/1 -> ADD_LKIN/7(OSEM_V1_In)
  Demux4/6 -> ADD_LKIN/6(LKIN_H3_In)
  Demux4/5 -> ADD_LKIN/5(LKIN_H2_In)
  Demux4/4 -> ADD_LKIN/4(LKIN_H1_In)
  Demux4/3 -> ADD_LKIN/3(LKIN_V3_In)
  Demux4/2 -> ADD_LKIN/2(LKN_V2_In)
  Demux4/1 -> ADD_LKIN/1(LKN_V1_In)
  ADD_LKIN/6(H3_Out) -> COILOUTF/6
  ADD_LKIN/5(H2_Out) -> COILOUTF/5
  ADD_LKIN/4(H1_Out) -> COILOUTF/4
  ADD_LKIN/3(V3_Out) -> COILOUTF/3
  ADD_LKIN/2(V2_Out) -> COILOUTF/2
  ADD_LKIN/1(V1_Out) -> COILOUTF/1
  Mux4/1 -> LKIN2OSEM/1
  LKIN2OSEM/1 -> Demux4/1
  LKIN/1(LKIN_P_Out) -> Mux4/1
  [LOCKSTATE] -> LOCK_STATE_Out/1
  LOCK/1(LOCK_STATE_Out) -> [LOCKSTATE]
  ADD/6(YAW_MAIN_Out) -> Mux3/6
  ADD/5(PITCH_MAIN_Out) -> Mux3/5
  ADD/4(ROLL_MAIN_Out) -> Mux3/4
  ADD/3(VERT_MAIN_Out) -> Mux3/3
  ADD/2(TRANS_MAIN_Out) -> Mux3/2
  ADD/1(LONG_MAIN_Out) -> Mux3/1
  [DAMPSTATE] -> DAMP_STATE_Out/1
  DAMP/7(DAMP_STATE_Out) -> [DAMPSTATE]
  [WDBLOCKFLAG] -> WD_BLOCK_Out/1
  Demux2/6 -> DAMP/6(YAW_In)
  Demux2/5 -> DAMP/5(PITCH_In)
  Demux2/4 -> DAMP/4(ROLL_In)
  Demux2/3 -> DAMP/3(VERT_In)
  Demux2/2 -> DAMP/2(TRANS_In)
  Demux2/1 -> DAMP/1(LONG_In)
  [WDBLOCKFLAG] -> MASTER/8(WDFLAG)
  Demux5/6 -> ISIWIT/6(YAW_In)
  Demux5/5 -> ISIWIT/5(PITCH_In)
  Demux5/4 -> ISIWIT/4(ROLL_In)
  Demux5/3 -> ISIWIT/3(VERT_In)
  Demux5/2 -> ISIWIT/2(TRANS_In)
  Demux5/1 -> ISIWIT/1(LONG_In)
  CART2EUL/1 -> Demux5/1
  Mux5/1 -> CART2EUL/1
  ISIINF/6(RY_Out) -> Mux5/6
  ISIINF/5(RX_Out) -> Mux5/5
  ISIINF/4(Z_Out) -> Mux5/4
  ISIINF/3(RZ_Out) -> Mux5/3
  ISIINF/2(Y_Out) -> Mux5/2
  ISIINF/1(X_Out) -> Mux5/1
  ISI_RY_In/1 -> ISIINF/6(RY_In)
  ISI_RX_In/1 -> ISIINF/5(RX_In)
  ISI_Z_In/1 -> ISIINF/4(Z_In)
  ISI_RZ_In/1 -> ISIINF/3(RZ_In)
  ISI_Y_In/1 -> ISIINF/2(Y_In)
  ISI_X_In/1 -> ISIINF/1(X_In)
  OSEMINF/6(H3_Out) -> Mux2/6
  OSEMINF/5(H2_Out) -> Mux2/5
  OSEMINF/4(H1_Out) -> Mux2/4
  OSEMINF/3(V3_Out) -> Mux2/3
  OSEMINF/2(V2_Out) -> Mux2/2
  OSEMINF/1(V1_Out) -> Mux2/1
  OSEM_V1_In/1 -> OSEMINF/1(V1_In), Bus Creator1/1
  OSEM_V2_In/1 -> OSEMINF/2(V2_In), Bus Creator1/2
  OSEM_V3_In/1 -> OSEMINF/3(V3_In), Bus Creator1/3
  OSEM_H1_In/1 -> OSEMINF/4(H1_In), Bus Creator1/4
  OSEM_H2_In/1 -> OSEMINF/5(H2_In), Bus Creator1/5
  OSEM_H3_In/1 -> OSEMINF/6(H3_In), Bus Creator1/6
  Mux2/1 -> OSEM2EUL/1
  ISC_LONG_In/1 -> LOCK/1(LONG_In)
  ISC_PITCH_In/1 -> LOCK/2(PITCH_In)
  ISC_YAW_In/1 -> LOCK/3(YAW_In)
  Bus Creator1/1 -> [OSEM2WD]
  [OSEM2WD] -> Bus Selector/1
  Bus Selector/1 -> WD/1(OSEM_V1_In)  "<OSEM_V1>"
  Bus Selector/2 -> WD/2(OSEM_V2_In)  "<OSEM_V2>"
  Bus Selector/3 -> WD/3(OSEM_V3_In)  "<OSEM_V3>"
  Bus Selector/4 -> WD/4(OSEM_H1_In)  "<OSEM_H1>"
  Bus Selector/5 -> WD/5(OSEM_H2_In)  "<OSEM_H2>"
  Bus Selector/6 -> WD/6(OSEM_H3_In)  "<OSEM_H3>"
  OSEM2EUL/1 -> Demux1/1
  Demux1/1 -> Mux1/1
  Demux1/2 -> Mux1/2
  Demux1/3 -> Mux1/3
  Demux1/4 -> Mux1/4
  Demux1/5 -> Mux1/5
  Demux1/6 -> Mux1/6
  Mux1/1 -> SENSALIGN/1
  SENSALIGN/1 -> Demux2/1
  MASTER/1(V1_Out) -> COIL_V1_Out/1
  MASTER/2(V2_Out) -> COIL_V2_Out/1
  MASTER/3(V3_Out) -> COIL_V3_Out/1
  MASTER/4(H1_Out) -> COIL_H1_Out/1
  MASTER/5(H2_Out) -> COIL_H2_Out/1
  MASTER/6(H3_Out) -> COIL_H3_Out/1
  Mux3/1 -> EUL2OSEM/1
  EUL2OSEM/1 -> Demux3/1
  Demux9/1 -> [WDBLOCKFLAG], WDMON/1(BLOCK_Flag)
  Demux9/2 -> WDMON/2(STATE_Flag)
  Demux9/3 -> WDMON/3(FIRST_Flag)
  Demux9/4 -> WDMON/4(CURRENT_Flag)
  COILOUTF/1 -> MASTER/1(F1_In)
  COILOUTF/2 -> MASTER/2(F2_In)
  COILOUTF/3 -> MASTER/3(F3_In)
  COILOUTF/4 -> MASTER/4(LF_In)
  COILOUTF/5 -> MASTER/5(RT_In)
  COILOUTF/6 -> MASTER/6(SD_In)
  Mux9/1 -> WATCHDOG/1
  WATCHDOG/1 -> Demux9/1
